simulink library "CTRL_TRGT_UG"  (R2023b)
settings: Solver=VariableStepAuto  StartTime=0.0  StopTime=10.0  RelTol=1e-3
undefined symbols (not defined in the file or in its folder): CTRL_TRGT_UG_p_SwtManUndStGra_na, p_TirCorStiFr_Nprad, p_TirCorStiRe_Nprad
settings Model: Creator=blatak  LastModifiedBy=blatak

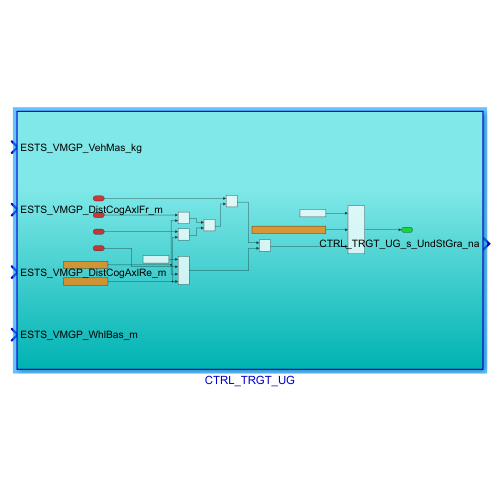
[thumbnail: Simulink's stored preview of the top-level diagram]
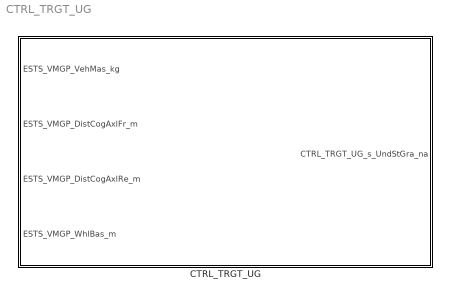
== system CTRL_TRGT_UG ==
  CTRL_TRGT_UG : Subsystem

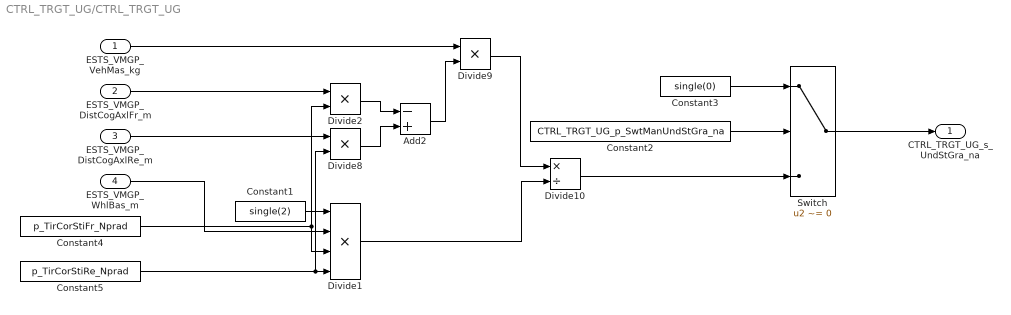
== system CTRL_TRGT_UG/CTRL_TRGT_UG ==
  ESTS_VMGP_VehMas_kg : Inport
  ESTS_VMGP_DistCogAxlFr_m : Inport  Port=2
  ESTS_VMGP_DistCogAxlRe_m : Inport  Port=3
  ESTS_VMGP_WhlBas_m : Inport  Port=4
  Add2 : Sum  Inputs=-+
  Constant1 : Constant  Value=single(2)
  Constant2 : Constant  Value=CTRL_TRGT_UG_p_SwtManUndStGra_na
  Constant3 : Constant  Value=single(0)
  Constant4 : Constant  Value=p_TirCorStiFr_Nprad
  Constant5 : Constant  Value=p_TirCorStiRe_Nprad
  Divide1 : Product  Inputs=****
  Divide10 : Product  Inputs=*/
  Divide2 : Product  Inputs=**
  Divide8 : Product  Inputs=**
  Divide9 : Product  Inputs=**
  Switch : Switch  Criteria=u2 ~= 0  SaturateOnIntegerOverflow=off  InputSameDT=off
  CTRL_TRGT_UG_s_UndStGra_na : Outport
  wires:
  Constant5/1 -> Divide8/2, Divide1/4
  Constant4/1 -> Divide1/3, Divide2/2
  ESTS_VMGP_WhlBas_m/1 -> Divide1/2
  Constant1/1 -> Divide1/1
  ESTS_VMGP_DistCogAxlFr_m/1 -> Divide2/1
  ESTS_VMGP_DistCogAxlRe_m/1 -> Divide8/1
  Divide8/1 -> Add2/2
  Divide2/1 -> Add2/1
  ESTS_VMGP_VehMas_kg/1 -> Divide9/1
  Add2/1 -> Divide9/2
  Divide9/1 -> Divide10/1
  Divide1/1 -> Divide10/2
  Constant2/1 -> Switch/2
  Switch/1 -> CTRL_TRGT_UG_s_UndStGra_na/1
  Divide10/1 -> Switch/3
  Constant3/1 -> Switch/1
